simulink library "dhp"  (R2021b)
settings: Solver=VariableStepAuto  StartTime=0.0  StopTime=10.0  RelTol=1e-3
undefined symbols (not defined in the file): ADHP_HysOffset_X_pct, ENUM_POWERSTA_OFF, ENUM_POWERSTA_STANDBY, ENUM_RANGESTA_12IN, ENUM_RANGESTA_12OUT, ENUM_RANGESTA_1OUT, ENUM_RANGESTA_2OUT, ENUM_RESETPEDALZEROPOSREQ_START, FALSE, HUNDRED, KDHP_AcceleratorLoadScalr_gain, KDHP_AccPedalDepressed_pct, KDHP_AccPedalReleased_pct, KDHP_ActAPSPosn_pct_ovrdflg, KDHP_ActAPSPosn_pct_ovrdval, KDHP_DeadBand_pct, KDHP_EAPS11OutWT_gain, KDHP_EAPS12Disagree_pct, KDHP_EAPS12DisagreeTime_s, KDHP_EAPS12OutWT_gain, KDHP_EAPS1AOutWT_gain, KDHP_EAPS1BADHigh_pct, KDHP_EAPS1BADLow_pct, KDHP_EAPS1BADTime_s, KDHP_EAPS1Min_pct_ovrdflg, KDHP_EAPS1Min_pct_ovrdval, KDHP_EAPS1MINInitLowLim_pct, KDHP_EAPS1MINInitUpLim_pct, KDHP_EAPS1WT_gain, KDHP_EAPS21OutWT_gain, KDHP_EAPS22OutWT_gain, KDHP_EAPS2AOutWT_gain, KDHP_EAPS2BADHigh_pct, KDHP_EAPS2BADLow_pct, KDHP_EAPS2BADTime_s, KDHP_EAPS2Min_pct_ovrdflg, KDHP_EAPS2Min_pct_ovrdval, KDHP_EAPS2MINInitLowLim_pct, KDHP_EAPS2MINInitUpLim_pct, KDHP_EAPS2Offset_pct, KDHP_EAPS2Scaler_gain, KDHP_EAPS2WT_gain, KDHP_EAPSCRBadWDSP_pct, KDHP_EAPSLearnDwHigh_pct, KDHP_EAPSLearnDwLow_pct, KDHP_EAPSLearnDwMAX_pct, KDHP_EAPSLearnUpHigh_pct, KDHP_EAPSLearnUpLow_pct, KDHP_EAPSLearnUpOffset_pct, KDHP_EAPSMINLowerLimit_pct, KDHP_EAPSStableThrsh_pct, KDHP_EAPSStableTime_s, KDHP_EPEDPOSNUpLimit_pct, KDHP_GetNRMBaseTime_s, KDHP_LVBattHigh_V, KDHP_LVBattHighLimit_V, KDHP_LVBattLow_V, MDHP_HysOffset_Y_pct, TRUE, ZERO_FLOAT
libraries: hcu_lib x6, simulink x4
(part 1 of 2)
settings Model: Creator=Shawn  LastModifiedBy=FVT23033
settings SolverCC: AlgebraicLoopSolver=TrustRegion

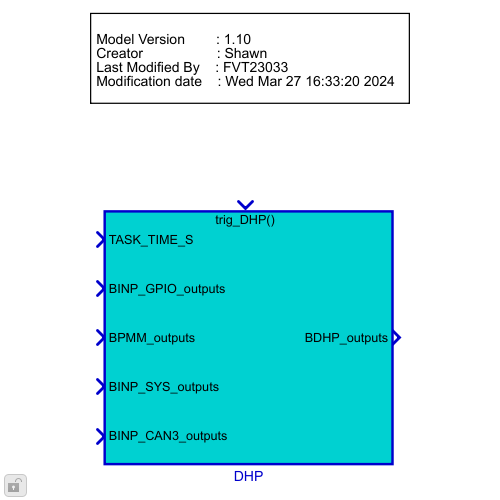
[thumbnail: Simulink's stored preview of the top-level diagram]
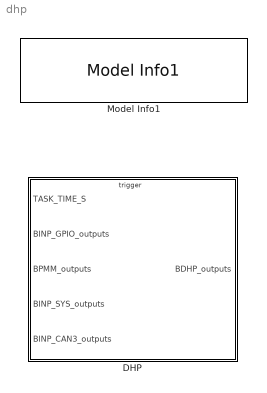
== system dhp ==
  DHP : Subsystem  TreatAsAtomicUnit=on
      settings: RTWSystemCode=Nonreusable function  RTWFcnNameOpts=Use subsystem name  RTWFileNameOpts=Use subsystem name
  Model Info1 : hcu_lib/Model Info1  BlockCM=None  Frame=on  DisplayStringWithTags=|  HorizontalTextAlignment=Left  LeftAlignmentValue=0.02  SourceBlockDiagram=hcu_lib  TagMaxNumber=20
      | Model Version        : %<ModelVersion>
      | Creator                   : %<Creator>
      | Last Modified By    : %<LastModifiedBy>
      | Modification date    : %<LastModificationDate>

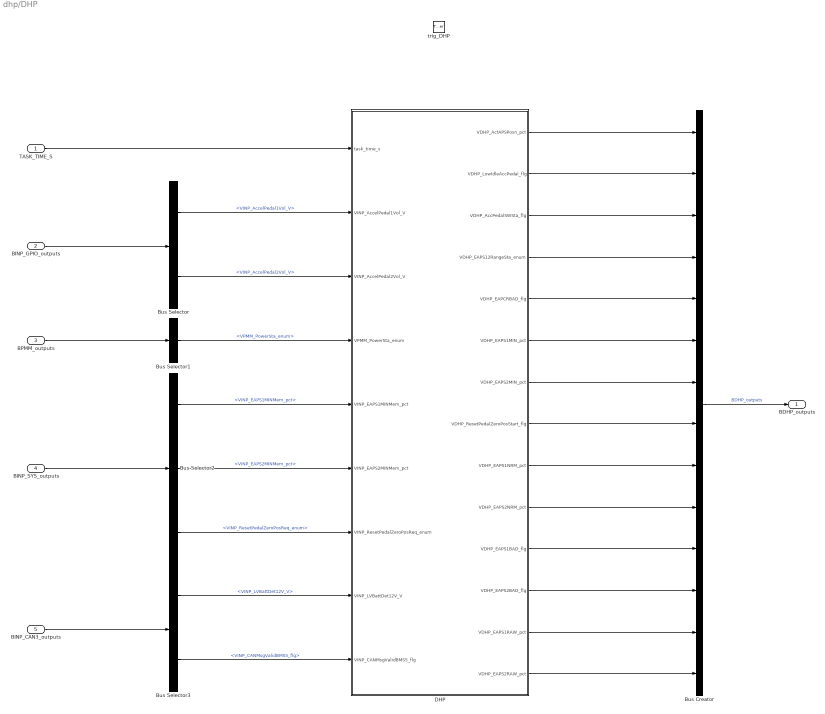
== system dhp/DHP ==
  TASK_TIME_S : Inport
  BINP_GPIO_outputs : Inport  Port=2  OutDataTypeStr=Bus: BINP_GPIO_outputs
  BPMM_outputs : Inport  Port=3  OutDataTypeStr=Bus: BPMM_outputs
  BINP_SYS_outputs : Inport  Port=4  OutDataTypeStr=Bus: BINP_SYS_outputs
  BINP_CAN3_outputs : Inport  Port=5  OutDataTypeStr=Bus: BINP_CAN3_outputs
  trig_DHP : TriggerPort  TriggerType=function-call  VariantControl=(inherit)
  Bus Creator : BusCreator  Inputs=14  OutDataTypeStr=Bus: BDHP_outputs  NonVirtualBus=on
  Bus Selector : BusSelector  OutputSignals=VINP_AccelPedal1Vol_V,VINP_AccelPedal2Vol_V
  Bus Selector1 : BusSelector  OutputSignals=VPMM_PowerSta_enum
  Bus Selector2 : BusSelector  OutputSignals=VINP_EAPS1MINMem_pct,VINP_EAPS2MINMem_pct,VINP_ResetPedalZeroPosReq_enum
  Bus Selector3 : BusSelector  OutputSignals=VINP_LVBattDet12V_V,VINP_CANMsgValidBMS5_flg
  DHP : Subsystem
  BDHP_outputs : Outport  OutDataTypeStr=Bus: BDHP_outputs  VectorParamsAs1DForOutWhenUnconnected=off
  wires:
  Bus Selector/1 -> DHP/2(VINP_AccelPedal1Vol_V)  "<VINP_AccelPedal1Vol_V>"
  BINP_GPIO_outputs/1 -> Bus Selector/1
  TASK_TIME_S/1 -> DHP/1(task_time_s)
  Bus Selector/2 -> DHP/3(VINP_AccelPedal2Vol_V)  "<VINP_AccelPedal2Vol_V>"
  Bus Creator/1 -> BDHP_outputs/1  "BDHP_outputs"
  DHP/1(VDHP_ActAPSPosn_pct) -> Bus Creator/1
  DHP/2(VDHP_LowIdleAccPedal_flg) -> Bus Creator/2
  BPMM_outputs/1 -> Bus Selector1/1
  Bus Selector1/1 -> DHP/4(VPMM_PowerSta_enum)  "<VPMM_PowerSta_enum>"
  DHP/3(VDHP_AccPedalSWSta_flg) -> Bus Creator/3
  DHP/4(VDHP_EAPS12RangeSta_enum) -> Bus Creator/4
  DHP/5(VDHP_EAPCRBAD_flg) -> Bus Creator/5
  DHP/6(VDHP_EAPS1MIN_pct) -> Bus Creator/6
  DHP/7(VDHP_EAPS2MIN_pct) -> Bus Creator/7
  BINP_SYS_outputs/1 -> Bus Selector2/1
  Bus Selector2/1 -> DHP/5(VINP_EAPS1MINMem_pct)  "<VINP_EAPS1MINMem_pct>"
  Bus Selector2/2 -> DHP/6(VINP_EAPS2MINMem_pct)  "<VINP_EAPS2MINMem_pct>"
  BINP_CAN3_outputs/1 -> Bus Selector3/1
  Bus Selector3/1 -> DHP/8(VINP_LVBattDet12V_V)  "<VINP_LVBattDet12V_V>"
  Bus Selector3/2 -> DHP/9(VINP_CANMsgValidBMS5_flg)  "<VINP_CANMsgValidBMS5_flg>"
  Bus Selector2/3 -> DHP/7(VINP_ResetPedalZeroPosReq_enum)  "<VINP_ResetPedalZeroPosReq_enum>"
  DHP/8(VDHP_ResetPedalZeroPosStart_flg) -> Bus Creator/8
  DHP/9(VDHP_EAPS1NRM_pct) -> Bus Creator/9
  DHP/10(VDHP_EAPS2NRM_pct) -> Bus Creator/10
  DHP/11(VDHP_EAPS1BAD_flg) -> Bus Creator/11
  DHP/12(VDHP_EAPS2BAD_flg) -> Bus Creator/12
  DHP/13(VDHP_EAPS1RAW_pct) -> Bus Creator/13
  DHP/14(VDHP_EAPS2RAW_pct) -> Bus Creator/14

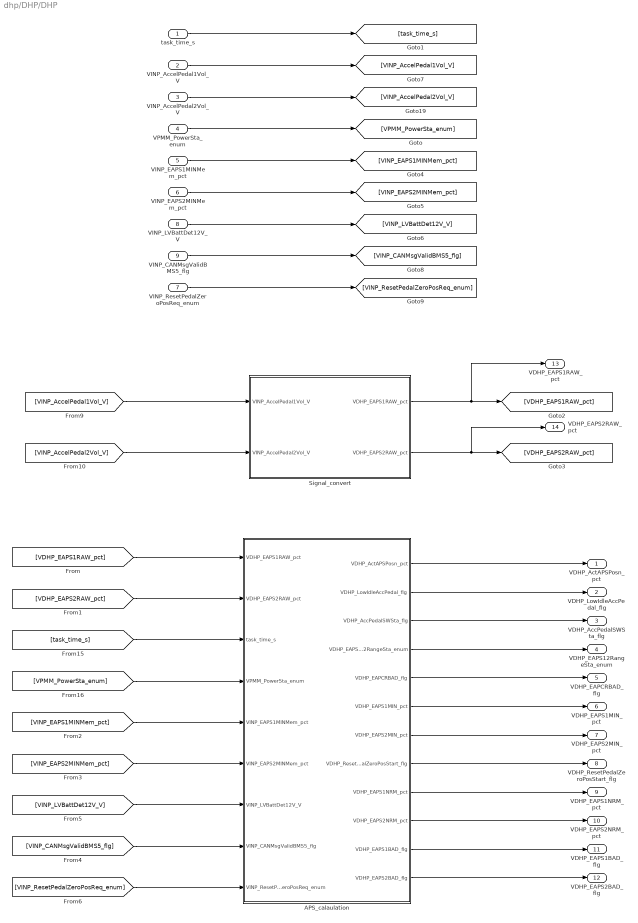
== system dhp/DHP/DHP ==
  task_time_s : Inport
  VINP_AccelPedal1Vol_V : Inport  Port=2
  VINP_AccelPedal2Vol_V : Inport  Port=3
  VPMM_PowerSta_enum : Inport  Port=4
  VINP_EAPS1MINMem_pct : Inport  Port=5
  VINP_EAPS2MINMem_pct : Inport  Port=6
  VINP_ResetPedalZeroPosReq_enum : Inport  Port=7
  VINP_LVBattDet12V_V : Inport  Port=8
  VINP_CANMsgValidBMS5_flg : Inport  Port=9
  APS_calaulation : Subsystem
  Signal_convert : Subsystem
  VDHP_ActAPSPosn_pct : Outport  VectorParamsAs1DForOutWhenUnconnected=off
  VDHP_LowIdleAccPedal_flg : Outport  Port=2  VectorParamsAs1DForOutWhenUnconnected=off
  VDHP_AccPedalSWSta_flg : Outport  Port=3  VectorParamsAs1DForOutWhenUnconnected=off
  VDHP_EAPS12RangeSta_enum : Outport  Port=4  VectorParamsAs1DForOutWhenUnconnected=off
  VDHP_EAPCRBAD_flg : Outport  Port=5  VectorParamsAs1DForOutWhenUnconnected=off
  VDHP_EAPS1MIN_pct : Outport  Port=6  VectorParamsAs1DForOutWhenUnconnected=off
  VDHP_EAPS2MIN_pct : Outport  Port=7  VectorParamsAs1DForOutWhenUnconnected=off
  VDHP_ResetPedalZeroPosStart_flg : Outport  Port=8  VectorParamsAs1DForOutWhenUnconnected=off
  VDHP_EAPS1NRM_pct : Outport  Port=9  VectorParamsAs1DForOutWhenUnconnected=off
  VDHP_EAPS2NRM_pct : Outport  Port=10  VectorParamsAs1DForOutWhenUnconnected=off
  VDHP_EAPS1BAD_flg : Outport  Port=11
  VDHP_EAPS2BAD_flg : Outport  Port=12
  VDHP_EAPS1RAW_pct : Outport  Port=13
  VDHP_EAPS2RAW_pct : Outport  Port=14
  wires:
  VPMM_PowerSta_enum/1 -> [VPMM_PowerSta_enum]
  task_time_s/1 -> [task_time_s]
  VINP_AccelPedal1Vol_V/1 -> [VINP_AccelPedal1Vol_V]
  VINP_AccelPedal2Vol_V/1 -> [VINP_AccelPedal2Vol_V]
  APS_calaulation/1(VDHP_ActAPSPosn_pct) -> VDHP_ActAPSPosn_pct/1
  APS_calaulation/2(VDHP_LowIdleAccPedal_flg) -> VDHP_LowIdleAccPedal_flg/1
  [VPMM_PowerSta_enum] -> APS_calaulation/4(VPMM_PowerSta_enum)
  [VINP_AccelPedal1Vol_V] -> Signal_convert/1(VINP_AccelPedal1Vol_V)
  [VINP_AccelPedal2Vol_V] -> Signal_convert/2(VINP_AccelPedal2Vol_V)
  Signal_convert/1(VDHP_EAPS1RAW_pct) -> VDHP_EAPS1RAW_pct/1, [VDHP_EAPS1RAW_pct]
  [VDHP_EAPS1RAW_pct] -> APS_calaulation/1(VDHP_EAPS1RAW_pct)
  Signal_convert/2(VDHP_EAPS2RAW_pct) -> VDHP_EAPS2RAW_pct/1, [VDHP_EAPS2RAW_pct]
  [VDHP_EAPS2RAW_pct] -> APS_calaulation/2(VDHP_EAPS2RAW_pct)
  APS_calaulation/3(VDHP_AccPedalSWSta_flg) -> VDHP_AccPedalSWSta_flg/1
  APS_calaulation/5(VDHP_EAPCRBAD_flg) -> VDHP_EAPCRBAD_flg/1
  APS_calaulation/4(VDHP_EAPS12RangeSta_enum) -> VDHP_EAPS12RangeSta_enum/1
  [task_time_s] -> APS_calaulation/3(task_time_s)
  APS_calaulation/6(VDHP_EAPS1MIN_pct) -> VDHP_EAPS1MIN_pct/1
  APS_calaulation/7(VDHP_EAPS2MIN_pct) -> VDHP_EAPS2MIN_pct/1
  VINP_EAPS1MINMem_pct/1 -> [VINP_EAPS1MINMem_pct]
  VINP_EAPS2MINMem_pct/1 -> [VINP_EAPS2MINMem_pct]
  [VINP_EAPS1MINMem_pct] -> APS_calaulation/5(VINP_EAPS1MINMem_pct)
  [VINP_EAPS2MINMem_pct] -> APS_calaulation/6(VINP_EAPS2MINMem_pct)
  VINP_CANMsgValidBMS5_flg/1 -> [VINP_CANMsgValidBMS5_flg]
  VINP_LVBattDet12V_V/1 -> [VINP_LVBattDet12V_V]
  [VINP_LVBattDet12V_V] -> APS_calaulation/7(VINP_LVBattDet12V_V)
  [VINP_CANMsgValidBMS5_flg] -> APS_calaulation/8(VINP_CANMsgValidBMS5_flg)
  VINP_ResetPedalZeroPosReq_enum/1 -> [VINP_ResetPedalZeroPosReq_enum]
  [VINP_ResetPedalZeroPosReq_enum] -> APS_calaulation/9(VINP_ResetPedalZeroPosReq_enum)
  APS_calaulation/8(VDHP_ResetPedalZeroPosStart_flg) -> VDHP_ResetPedalZeroPosStart_flg/1
  APS_calaulation/9(VDHP_EAPS1NRM_pct) -> VDHP_EAPS1NRM_pct/1
  APS_calaulation/10(VDHP_EAPS2NRM_pct) -> VDHP_EAPS2NRM_pct/1
  APS_calaulation/12(VDHP_EAPS2BAD_flg) -> VDHP_EAPS2BAD_flg/1
  APS_calaulation/11(VDHP_EAPS1BAD_flg) -> VDHP_EAPS1BAD_flg/1

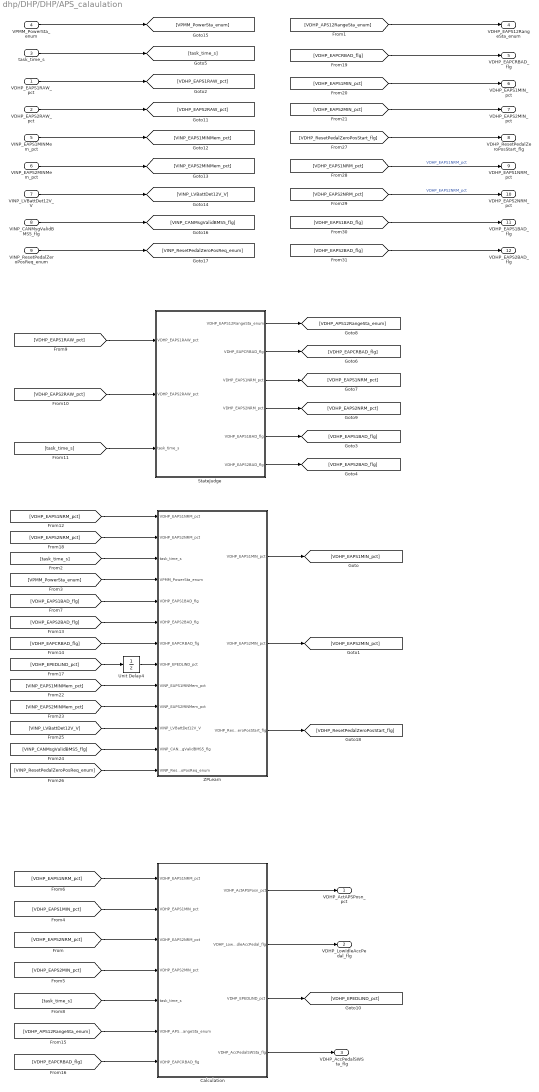
== system dhp/DHP/DHP/APS_calaulation ==
  VDHP_EAPS1RAW_pct : Inport
  VDHP_EAPS2RAW_pct : Inport  Port=2
  task_time_s : Inport  Port=3
  VPMM_PowerSta_enum : Inport  Port=4
  VINP_EAPS1MINMem_pct : Inport  Port=5
  VINP_EAPS2MINMem_pct : Inport  Port=6
  VINP_LVBattDet12V_V : Inport  Port=7
  VINP_CANMsgValidBMS5_flg : Inport  Port=8
  VINP_ResetPedalZeroPosReq_enum : Inport  Port=9
  Calculation : Subsystem
  StateJudge : Subsystem
  Unit Delay4 : UnitDelay  SampleTime=-1  HasFrameUpgradeWarning=on
  ZPLearn : Subsystem
  VDHP_ActAPSPosn_pct : Outport
  VDHP_LowIdleAccPedal_flg : Outport  Port=2
  VDHP_AccPedalSWSta_flg : Outport  Port=3
  VDHP_EAPS12RangeSta_enum : Outport  Port=4
  VDHP_EAPCRBAD_flg : Outport  Port=5
  VDHP_EAPS1MIN_pct : Outport  Port=6
  VDHP_EAPS2MIN_pct : Outport  Port=7
  VDHP_ResetPedalZeroPosStart_flg : Outport  Port=8
  VDHP_EAPS1NRM_pct : Outport  Port=9
  VDHP_EAPS2NRM_pct : Outport  Port=10
  VDHP_EAPS1BAD_flg : Outport  Port=11
  VDHP_EAPS2BAD_flg : Outport  Port=12
  wires:
  [VDHP_EAPS1MIN_pct] -> Calculation/2(VDHP_EAPS1MIN_pct)
  StateJudge/4(VDHP_EAPS2NRM_pct) -> [VDHP_EAPS2NRM_pct]
  [VDHP_EAPS1BAD_flg] -> ZPLearn/5(VDHP_EAPS1BAD_flg)
  [VDHP_EAPS2NRM_pct] -> Calculation/3(VDHP_EAPS2NRM_pct)
  [VDHP_EAPS1RAW_pct] -> StateJudge/1(VDHP_EAPS1RAW_pct)
  VDHP_EAPS2RAW_pct/1 -> [VDHP_EAPS2RAW_pct]
  [VPMM_PowerSta_enum] -> ZPLearn/4(VPMM_PowerSta_enum)
  [task_time_s] -> ZPLearn/3(task_time_s)
  [VDHP_EAPS2MIN_pct] -> Calculation/4(VDHP_EAPS2MIN_pct)
  [task_time_s] -> Calculation/5(task_time_s)
  StateJudge/1(VDHP_EAPS12RangeSta_enum) -> [VDHP_APS12RangeSta_enum]
  [VDHP_EAPS2NRM_pct] -> ZPLearn/2(VDHP_EAPS2NRM_pct)
  VPMM_PowerSta_enum/1 -> [VPMM_PowerSta_enum]
  VDHP_EAPS1RAW_pct/1 -> [VDHP_EAPS1RAW_pct]
  [VDHP_EAPS1NRM_pct] -> ZPLearn/1(VDHP_EAPS1NRM_pct)
  StateJudge/5(VDHP_EAPS1BAD_flg) -> [VDHP_EAPS1BAD_flg]
  [VDHP_EAPS1NRM_pct] -> Calculation/1(VDHP_EAPS1NRM_pct)
  task_time_s/1 -> [task_time_s]
  ZPLearn/2(VDHP_EAPS2MIN_pct) -> [VDHP_EAPS2MIN_pct]
  ZPLearn/1(VDHP_EAPS1MIN_pct) -> [VDHP_EAPS1MIN_pct]
  [VDHP_APS12RangeSta_enum] -> Calculation/6(VDHP_APS12RangeSta_enum)
  [VDHP_EAPCRBAD_flg] -> ZPLearn/7(VDHP_EAPCRBAD_flg)
  [VDHP_EAPS2RAW_pct] -> StateJudge/2(VDHP_EAPS2RAW_pct)
  Calculation/1(VDHP_ActAPSPosn_pct) -> VDHP_ActAPSPosn_pct/1
  [VDHP_EAPCRBAD_flg] -> Calculation/7(VDHP_EAPCRBAD_flg)
  StateJudge/3(VDHP_EAPS1NRM_pct) -> [VDHP_EAPS1NRM_pct]
  StateJudge/2(VDHP_EAPCRBAD_flg) -> [VDHP_EAPCRBAD_flg]
  [VDHP_EAPS2BAD_flg] -> ZPLearn/6(VDHP_EAPS2BAD_flg)
  StateJudge/6(VDHP_EAPS2BAD_flg) -> [VDHP_EAPS2BAD_flg]
  [task_time_s] -> StateJudge/3(task_time_s)
  Calculation/2(VDHP_LowIdleAccPedal_flg) -> VDHP_LowIdleAccPedal_flg/1
  Calculation/3(VDHP_EPEDLIND_pct) -> [VDHP_EPEDLIND_pct]
  [VDHP_EPEDLIND_pct] -> Unit Delay4/1
  Unit Delay4/1 -> ZPLearn/8(VDHP_EPEDLIND_pct)
  Calculation/4(VDHP_AccPedalSWSta_flg) -> VDHP_AccPedalSWSta_flg/1
  [VDHP_EAPCRBAD_flg] -> VDHP_EAPCRBAD_flg/1
  [VDHP_APS12RangeSta_enum] -> VDHP_EAPS12RangeSta_enum/1
  [VDHP_EAPS1MIN_pct] -> VDHP_EAPS1MIN_pct/1
  [VDHP_EAPS2MIN_pct] -> VDHP_EAPS2MIN_pct/1
  VINP_EAPS1MINMem_pct/1 -> [VINP_EAPS1MINMem_pct]
  VINP_EAPS2MINMem_pct/1 -> [VINP_EAPS2MINMem_pct]
  [VINP_EAPS1MINMem_pct] -> ZPLearn/9(VINP_EAPS1MINMem_pct)
  [VINP_EAPS2MINMem_pct] -> ZPLearn/10(VINP_EAPS2MINMem_pct)
  VINP_CANMsgValidBMS5_flg/1 -> [VINP_CANMsgValidBMS5_flg]
  VINP_LVBattDet12V_V/1 -> [VINP_LVBattDet12V_V]
  [VINP_LVBattDet12V_V] -> ZPLearn/11(VINP_LVBattDet12V_V)
  [VINP_CANMsgValidBMS5_flg] -> ZPLearn/12(VINP_CANMsgValidBMS5_flg)
  VINP_ResetPedalZeroPosReq_enum/1 -> [VINP_ResetPedalZeroPosReq_enum]
  [VINP_ResetPedalZeroPosReq_enum] -> ZPLearn/13(VINP_ResetPedalZeroPosReq_enum)
  ZPLearn/3(VDHP_ResetPedalZeroPosStart_flg) -> [VDHP_ResetPedalZeroPosStart_flg]
  [VDHP_ResetPedalZeroPosStart_flg] -> VDHP_ResetPedalZeroPosStart_flg/1
  [VDHP_EAPS1NRM_pct] -> VDHP_EAPS1NRM_pct/1  "VDHP_EAPS1NRM_pct"
  [VDHP_EAPS2NRM_pct] -> VDHP_EAPS2NRM_pct/1  "VDHP_EAPS2NRM_pct"
  [VDHP_EAPS1BAD_flg] -> VDHP_EAPS1BAD_flg/1
  [VDHP_EAPS2BAD_flg] -> VDHP_EAPS2BAD_flg/1

== system dhp/DHP/DHP/Signal_convert ==
  VINP_AccelPedal1Vol_V : Inport
  VINP_AccelPedal2Vol_V : Inport  Port=2
  1-D Lookup Table1 : Lookup_n-D  NumberOfTableDimensions=1  BreakpointsForDimension1=[0 5]  Table=[0 1]  ExtrapMethod=Clip  InternalRulePriority=Speed  RndMeth=Simplest  InputSameDT=on
  1-D Lookup Table4 : Lookup_n-D  NumberOfTableDimensions=1  BreakpointsForDimension1=[0 5]  Table=[0 1]  ExtrapMethod=Clip  InternalRulePriority=Speed  RndMeth=Simplest  InputSameDT=on
  Data Type Conversion : DataTypeConversion  OutDataTypeStr=single
  Data Type Conversion1 : DataTypeConversion  OutDataTypeStr=single
  Gain : Gain  Gain=HUNDRED
  Gain1 : Gain  Gain=HUNDRED
  VDHP_EAPS1RAW_pct : Outport
  VDHP_EAPS2RAW_pct : Outport  Port=2
  wires:
  VINP_AccelPedal1Vol_V/1 -> 1-D Lookup Table4/1
  VINP_AccelPedal2Vol_V/1 -> 1-D Lookup Table1/1
  Gain1/1 -> Data Type Conversion/1
  Data Type Conversion/1 -> VDHP_EAPS1RAW_pct/1  "VDHP_EAPS1RAW_pct"
  1-D Lookup Table4/1 -> Gain1/1
  Data Type Conversion1/1 -> VDHP_EAPS2RAW_pct/1  "VDHP_EAPS2RAW_pct"
  Gain/1 -> Data Type Conversion1/1
  1-D Lookup Table1/1 -> Gain/1

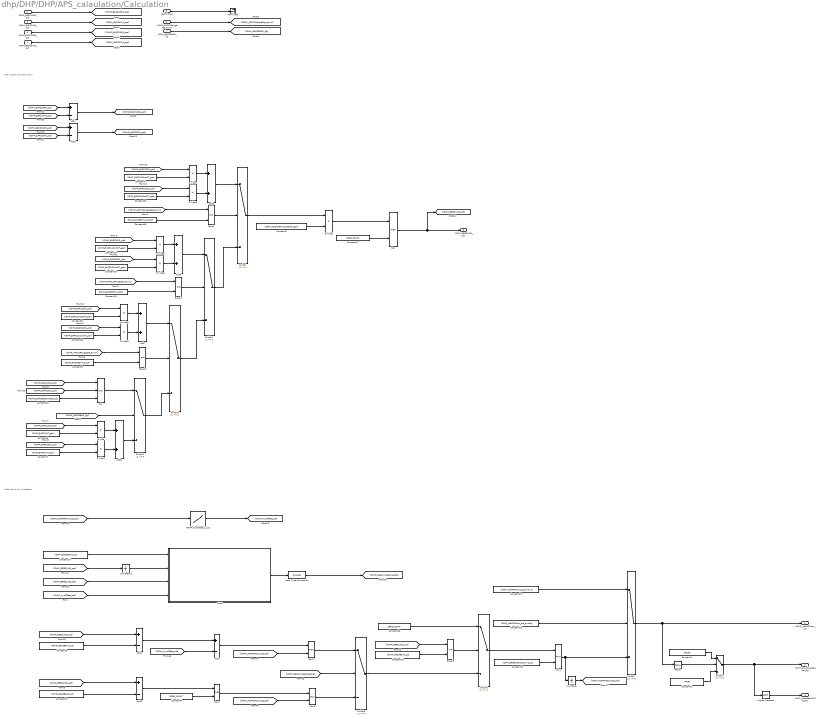
== system dhp/DHP/DHP/APS_calaulation/Calculation ==
  note: Dead band ans Hysteresis
  note: APS weight and calaulation
  VDHP_EAPS1NRM_pct : Inport
  VDHP_EAPS1MIN_pct : Inport  Port=2
  VDHP_EAPS2NRM_pct : Inport  Port=3
  VDHP_EAPS2MIN_pct : Inport  Port=4
  task_time_s : Inport  Port=5
  VDHP_APS12RangeSta_enum : Inport  Port=6
  VDHP_EAPCRBAD_flg : Inport  Port=7
  Add{1..4,6} (5 alike) : Sum  Inputs=+-
  Add{5,7..9} (4 alike) : Sum
  Chart : Stateflow chart  TreatAsAtomicUnit=on
  Constant1 : Constant  Value=FALSE
  Constant{9..10,13..14} (4 alike) : Constant  Value=KDHP_DeadBand_pct
  Constant11 : Constant  Value=ENUM_RANGESTA_1OUT
  Constant12 : Constant  Value=KDHP_EPEDPOSNUpLimit_pct
  Constant15 : Constant  Value=ZERO_FLOAT
  Constant16 : Constant  Value=KDHP_ActAPSPosn_pct_ovrdflg
  Constant17 : Constant  Value=ZERO_FLOAT
  Constant18 : Constant  Value=ENUM_RANGESTA_12OUT
  Constant19 : Constant  Value=KDHP_ActAPSPosn_pct_ovrdval
  Constant2 : Constant  Value=TRUE
  Constant20 : Constant  Value=KDHP_EAPSCRBadWDSP_pct
  Constant21 : Constant  Value=KDHP_EAPS12OutWT_gain
  Constant22 : Constant  Value=KDHP_EAPS22OutWT_gain
  Constant23 : Constant  Value=KDHP_EAPS11OutWT_gain
  Constant24 : Constant  Value=KDHP_EAPS21OutWT_gain
  Constant25 : Constant  Value=KDHP_EAPS2AOutWT_gain
  Constant3 : Constant  Value=KDHP_AcceleratorLoadScalr_gain
  Constant4 : Constant  Value=KDHP_EAPS1AOutWT_gain
  Constant5 : Constant  Value=ENUM_RANGESTA_2OUT
  Constant6 : Constant  Value=KDHP_EAPS1WT_gain
  Constant7 : Constant  Value=KDHP_EAPS2WT_gain
  Constant8 : Constant  Value=ZERO_FLOAT
  Data Type Conversion : DataTypeConversion  OutDataTypeStr=boolean
  Divide{,1..8} (9 alike) : Product  Inputs=**
  Equal : RelationalOperator  Operator===  OutDataTypeStr=boolean  RndMeth=Simplest
  Equal1 : RelationalOperator  Operator===  OutDataTypeStr=boolean  RndMeth=Simplest
  Equal2 : RelationalOperator  Operator===  OutDataTypeStr=boolean  RndMeth=Simplest
  Equal3 : RelationalOperator  Operator=<=  OutDataTypeStr=boolean  RndMeth=Simplest
  Logical Operator : Logic  Operator=NOT  AllPortsSameDT=off  OutDataTypeStr=boolean
  MDHP_HysOffset_Y_pct : Lookup_n-D  NumberOfTableDimensions=1  BreakpointsForDimension1=ADHP_HysOffset_X_pct  Table=MDHP_HysOffset_Y_pct  ExtrapMethod=Clip  InternalRulePriority=Speed  RndMeth=Simplest  InputSameDT=on
  Max : MinMax  Function=max  Inputs=2
  Max2 : MinMax  Function=max  Inputs=2
  Max3 : MinMax  Inputs=2
  Max4 : MinMax  Function=max  Inputs=2
  Min : MinMax  Inputs=3
  Min1 : MinMax  Inputs=2
  Relay : Relay  OnSwitchValue=KDHP_AccPedalDepressed_pct  OffSwitchValue=KDHP_AccPedalReleased_pct
      settings: AttributesFormatString=<ON = %<OnSwitchValue>>\n<OFF = %<OffSwitchValue>>
  Switch{,1..7} (8 alike) : Switch  Criteria=u2 ~= 0
      Switch1 settings: AttributesFormatString=<%<Criteria>>
  Terminator : Terminator
  Unit Delay : UnitDelay  SampleTime=-1  HasFrameUpgradeWarning=on
  Unit Delay1 : UnitDelay  SampleTime=-1  HasFrameUpgradeWarning=on
  VDHP_ActAPSPosn_pct : Outport
  VDHP_LowIdleAccPedal_flg : Outport  Port=2
  VDHP_EPEDLIND_pct : Outport  Port=3
  VDHP_AccPedalSWSta_flg : Outport  Port=4
  wires:
  Max/1 -> VDHP_EPEDLIND_pct/1, [VDHP_EPEDLIND_pct]  "VDHP_EPEDLIND_pct"
  VDHP_EAPS1NRM_pct/1 -> [VDHP_EAPS1NRM_pct]  "VDHP_EAPS1NRM_pct"
  VDHP_EAPS2NRM_pct/1 -> [VDHP_EAPS2NRM_pct]  "VDHP_EAPS2NRM_pct"
  VDHP_EAPS1MIN_pct/1 -> [VDHP_EAPS1MIN_pct]  "VDHP_EAPS1MIN_pct"
  VDHP_EAPS2MIN_pct/1 -> [VDHP_EAPS2MIN_pct]  "VDHP_EAPS2MIN_pct"
  task_time_s/1 -> Terminator/1  "task_time_s"
  VDHP_APS12RangeSta_enum/1 -> [VDHP_APS12RangeSta_enum]  "VDHP_APS12RangeSta_enum"
  VDHP_EAPCRBAD_flg/1 -> [VDHP_EAPCRBAD_flg]  "VDHP_EAPCRBAD_flg"
  Constant2/1 -> Switch1/3
  Switch1/1 -> Logical Operator/1, VDHP_LowIdleAccPedal_flg/1  "VDHP_LowIdleAccPedal_flg"
  Constant1/1 -> Switch1/1
  Relay/1 -> Switch1/2
  Constant3/1 -> Divide2/2
  Equal/1 -> Switch/2
  [VDHP_APS12RangeSta_enum] -> Equal/1
  Constant18/1 -> Equal/2
  Constant11/1 -> Equal1/2
  [VDHP_APS12RangeSta_enum] -> Equal1/1
  Equal1/1 -> Switch2/2
  Switch2/1 -> Switch/3
  [VDHP_EAPS2NRM_pct] -> Add3/1
  [VDHP_EAPS2MIN_pct] -> Add3/2
  Add3/1 -> [VDHP_EAPS2DIS_pct]  "VDHP_EAPS2DIS_pct"
  [VDHP_EAPS1NRM_pct] -> Add4/1
  Add4/1 -> [VDHP_EAPS1DIS_pct]  "VDHP_EAPS1DIS_pct"
  [VDHP_EAPS1MIN_pct] -> Add4/2
  Switch3/1 -> Switch2/3
  [VDHP_APS12RangeSta_enum] -> Equal2/1
  Constant5/1 -> Equal2/2
  Equal2/1 -> Switch3/2
  Switch4/1 -> Switch3/3
  [VDHP_EAPCRBAD_flg] -> Switch4/2
  Min/1 -> Switch4/1
  [VDHP_EAPS2DIS_pct] -> Min/2
  [VDHP_EAPS1DIS_pct] -> Min/1
  [VDHP_EAPS2DIS_pct] -> Divide1/1
  Divide1/1 -> Add5/2
  Divide/1 -> Add5/1
  Add5/1 -> Switch4/3
  [VDHP_EAPS1DIS_pct] -> Divide/1
  Constant6/1 -> Divide/2
  Constant7/1 -> Divide1/2
  Switch/1 -> Divide2/1  "VDHP_EAPSWDSP_pct"
  Constant12/1 -> Min1/2
  Switch7/1 -> VDHP_ActAPSPosn_pct/1, Relay/1  "VDHP_ActAPSPosn_pct"
  Divide2/1 -> Max/1
  Constant17/1 -> Max/2
  [VDHP_ActAPSPosnLast_pct] -> MDHP_HysOffset_Y_pct/1
  [VDHP_PedalIncreasing_flg] -> Switch5/2
  MDHP_HysOffset_Y_pct/1 -> [VDHP_HysOffset_pct]  "VDHP_HysOffset_pct"
  [VDHP_EPEDLIND_pct] -> Add1/1
  [VDHP_ActAPSPosnLast_pct] -> Max2/2
  Max2/1 -> Switch5/1
  Max4/1 -> Max3/1
  [VDHP_HysOffset_pct] -> Add2/2
  Add2/1 -> Max2/1
  [VDHP_ActAPSPosnLast_pct] -> Max3/2
  Max3/1 -> Switch5/3
  Add1/1 -> Add2/1
  [VDHP_EPEDLIND_pct] -> Add6/1
  Constant13/1 -> Add6/2
  Constant8/1 -> Max4/2
  Constant9/1 -> Add1/2
  Add6/1 -> Max4/1
  Unit Delay1/1 -> Chart/2(VDHP_EPEDLINDLast_pct)
  [VDHP_EPEDLIND_pct] -> Unit Delay1/1
  Chart/1(VDHP_PedalIncreasing_flg) -> Data Type Conversion/1
  Constant14/1 -> Chart/1(KDHP_DeadBand_pct)
  [VDHP_HysOffset_pct] -> Chart/4(VDHP_HysOffset_pct)
  [VDHP_EPEDLIND_pct] -> Chart/3(VDHP_EPEDLIND_pct)
  Data Type Conversion/1 -> [VDHP_PedalIncreasing_flg]  "VDHP_PedalIncreasing_flg"
  Switch5/1 -> Switch6/3
  Constant10/1 -> Equal3/2
  [VDHP_EPEDLIND_pct] -> Equal3/1
  Equal3/1 -> Switch6/2
  Constant15/1 -> Switch6/1
  Switch6/1 -> Min1/1
  Logical Operator/1 -> VDHP_AccPedalSWSta_flg/1  "VDHP_AccPedalSWSta_flg"
  Min1/1 -> Unit Delay/1, Switch7/3
  Constant16/1 -> Switch7/2
  Constant19/1 -> Switch7/1
  Unit Delay/1 -> [VDHP_ActAPSPosnLast_pct]
  Constant20/1 -> Min/3
  [VDHP_EAPS2DIS_pct] -> Divide4/1
  Constant22/1 -> Divide4/2
  Constant21/1 -> Divide3/2
  [VDHP_EAPS1DIS_pct] -> Divide3/1
  Divide4/1 -> Add7/2
  Divide3/1 -> Add7/1
  Add7/1 -> Switch3/1
  Divide5/1 -> Add8/1
  Constant24/1 -> Divide6/2
  Constant23/1 -> Divide5/2
  [VDHP_EAPS2DIS_pct] -> Divide6/1
  Divide6/1 -> Add8/2
  [VDHP_EAPS1DIS_pct] -> Divide5/1
  Add8/1 -> Switch2/1
  Add9/1 -> Switch/1
  [VDHP_EAPS1DIS_pct] -> Divide7/1
  [VDHP_EAPS2DIS_pct] -> Divide8/1
  Constant25/1 -> Divide8/2
  Constant4/1 -> Divide7/2
  Divide8/1 -> Add9/2
  Divide7/1 -> Add9/1

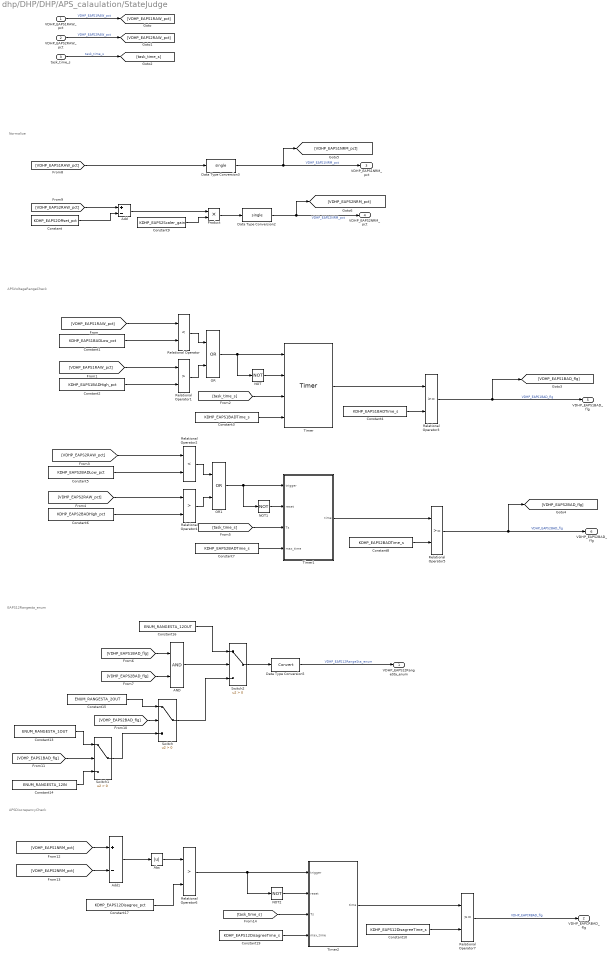
== system dhp/DHP/DHP/APS_calaulation/StateJudge ==
  note: APSDiscrepancyCheck
  note: EAPS12Rangesta_enum
  note: Normalize
  note: APSVoltageRangeCheck
  VDHP_EAPS1RAW_pct : Inport
  VDHP_EAPS2RAW_pct : Inport  Port=2
  task_time_s : Inport  Port=3
  AND : Logic  AllPortsSameDT=off  OutDataTypeStr=boolean
  Abs : Abs
  Add : Sum  Inputs=+-
  Add1 : Sum  Inputs=+-
  Constant : Constant  Value=KDHP_EAPS2Offset_pct
  Constant1 : Constant  Value=KDHP_EAPS1BADLow_pct
  Constant10 : Constant  Value=KDHP_EAPS12DisagreeTime_s
  Constant13 : Constant  Value=ENUM_RANGESTA_1OUT
  Constant14 : Constant  Value=ENUM_RANGESTA_12IN
  Constant15 : Constant  Value=ENUM_RANGESTA_2OUT
  Constant16 : Constant  Value=ENUM_RANGESTA_12OUT
  Constant17 : Constant  Value=KDHP_EAPS12Disagree_pct
  Constant19 : Constant  Value=KDHP_EAPS12DisagreeTime_s
  Constant2 : Constant  Value=KDHP_EAPS1BADHigh_pct
  Constant3 : Constant  Value=KDHP_EAPS1BADTime_s
  Constant4 : Constant  Value=KDHP_EAPS1BADTime_s
  Constant5 : Constant  Value=KDHP_EAPS2BADLow_pct
  Constant6 : Constant  Value=KDHP_EAPS2BADHigh_pct
  Constant7 : Constant  Value=KDHP_EAPS2BADTime_s
  Constant8 : Constant  Value=KDHP_EAPS2BADTime_s
  Constant9 : Constant  Value=KDHP_EAPS2Scaler_gain
  Data Type Conversion2 : DataTypeConversion  OutDataTypeStr=single
  Data Type Conversion3 : DataTypeConversion  OutDataTypeStr=single
  Data Type Conversion5 : DataTypeConversion
  NOT : Logic  Operator=NOT  AllPortsSameDT=off  OutDataTypeStr=boolean
  NOT1 : Logic  Operator=NOT  AllPortsSameDT=off  OutDataTypeStr=boolean
  NOT2 : Logic  Operator=NOT  AllPortsSameDT=off  OutDataTypeStr=boolean
  OR : Logic  Operator=OR  AllPortsSameDT=off  OutDataTypeStr=boolean
  OR1 : Logic  Operator=OR  AllPortsSameDT=off  OutDataTypeStr=boolean
  Product : Product
  Relational Operator : RelationalOperator  Operator=<  OutDataTypeStr=boolean  RndMeth=Simplest
  Relational Operator1 : RelationalOperator  Operator=>  OutDataTypeStr=boolean  RndMeth=Simplest
  Relational Operator2 : RelationalOperator  Operator=<  OutDataTypeStr=boolean  RndMeth=Simplest
  Relational Operator3 : RelationalOperator  OutDataTypeStr=boolean  RndMeth=Simplest
  Relational Operator4 : RelationalOperator  Operator=>  OutDataTypeStr=boolean  RndMeth=Simplest
  Relational Operator5 : RelationalOperator  OutDataTypeStr=boolean  RndMeth=Simplest
  Relational Operator6 : RelationalOperator  Operator=>  OutDataTypeStr=boolean  RndMeth=Simplest
  Relational Operator7 : RelationalOperator  OutDataTypeStr=boolean  RndMeth=Simplest
  Switch : Switch  Criteria=u2 > Threshold
  Switch1 : Switch  Criteria=u2 > Threshold
  Switch2 : Switch  Criteria=u2 > Threshold
  Timer : hcu_lib/Basic_Blocks/Timer
  Timer1 : Subsystem  mask(Timer){}
      mask help: Timer funcion.
  Timer2 : Subsystem  mask(Timer){}
      mask help: Timer funcion.
  VDHP_EAPS12RangeSta_enum : Outport
  VDHP_EAPCRBAD_flg : Outport  Port=2
  VDHP_EAPS1NRM_pct : Outport  Port=3
  VDHP_EAPS2NRM_pct : Outport  Port=4
  VDHP_EAPS1BAD_flg : Outport  Port=5
  VDHP_EAPS2BAD_flg : Outport  Port=6
  wires:
  Relational Operator1/1 -> OR/2
  [VDHP_EAPS1RAW_pct] -> Relational Operator1/1
  Relational Operator/1 -> OR/1
  VDHP_EAPS1RAW_pct/1 -> [VDHP_EAPS1RAW_pct]  "VDHP_EAPS1RAW_pct"
  [VDHP_EAPS1RAW_pct] -> Relational Operator/1
  VDHP_EAPS2RAW_pct/1 -> [VDHP_EAPS2RAW_pct]  "VDHP_EAPS2RAW_pct"
  task_time_s/1 -> [task_time_s]  "task_time_s"
  OR/1 -> NOT/1, Timer/1
  NOT/1 -> Timer/2
  Constant4/1 -> Relational Operator3/2
  Relational Operator3/1 -> VDHP_EAPS1BAD_flg/1, [VDHP_EAPS1BAD_flg]  "VDHP_EAPS1BAD_flg"
  Relational Operator5/1 -> VDHP_EAPS2BAD_flg/1, [VDHP_EAPS2BAD_flg]  "VDHP_EAPS2BAD_flg"
  Constant8/1 -> Relational Operator5/2
  OR1/1 -> Timer1/1(trigger), NOT1/1
  [VDHP_EAPS2RAW_pct] -> Relational Operator2/1
  Relational Operator2/1 -> OR1/1
  Constant5/1 -> Relational Operator2/2
  [VDHP_EAPS2RAW_pct] -> Relational Operator4/1
  Constant6/1 -> Relational Operator4/2
  Relational Operator4/1 -> OR1/2
  Constant1/1 -> Relational Operator/2
  Constant2/1 -> Relational Operator1/2
  [VDHP_EAPS1BAD_flg] -> AND/1
  [VDHP_EAPS2BAD_flg] -> AND/2
  Constant/1 -> Add/2
  Data Type Conversion2/1 -> [VDHP_EAPS2NRM_pct], VDHP_EAPS2NRM_pct/1  "VDHP_EAPS2NRM_pct"
  [VDHP_EAPS2BAD_flg] -> Switch/2
  Switch1/1 -> Switch/3
  [VDHP_EAPS1BAD_flg] -> Switch1/2
  AND/1 -> Switch2/2
  Switch/1 -> Switch2/3
  Constant13/1 -> Switch1/1
  Constant14/1 -> Switch1/3
  Constant15/1 -> Switch/1
  Switch2/1 -> Data Type Conversion5/1
  Constant16/1 -> Switch2/1
  [VDHP_EAPS1RAW_pct] -> Data Type Conversion3/1
  Data Type Conversion3/1 -> [VDHP_EAPS1NRM_pct], VDHP_EAPS1NRM_pct/1  "VDHP_EAPS1NRM_pct"
  [VDHP_EAPS1NRM_pct] -> Add1/1
  [VDHP_EAPS2NRM_pct] -> Add1/2
  Add1/1 -> Abs/1
  Abs/1 -> Relational Operator6/1
  Constant17/1 -> Relational Operator6/2
  Data Type Conversion5/1 -> VDHP_EAPS12RangeSta_enum/1  "VDHP_EAPS12RangeSta_enum"
  [VDHP_EAPS2RAW_pct] -> Add/1
  Add/1 -> Product/1
  Product/1 -> Data Type Conversion2/1
  Constant9/1 -> Product/2
  [task_time_s] -> Timer/3
  Timer/1 -> Relational Operator3/1
  Constant3/1 -> Timer/4
  NOT1/1 -> Timer1/2(reset)
  [task_time_s] -> Timer1/3(Ts)
  Constant7/1 -> Timer1/4(max_time)
  Timer1/1(time) -> Relational Operator5/1
  Relational Operator6/1 -> NOT2/1, Timer2/1(trigger)
  NOT2/1 -> Timer2/2(reset)
  [task_time_s] -> Timer2/3(Ts)
  Constant19/1 -> Timer2/4(max_time)
  Timer2/1(time) -> Relational Operator7/1
  Constant10/1 -> Relational Operator7/2
  Relational Operator7/1 -> VDHP_EAPCRBAD_flg/1  "VDHP_EAPCRBAD_flg"

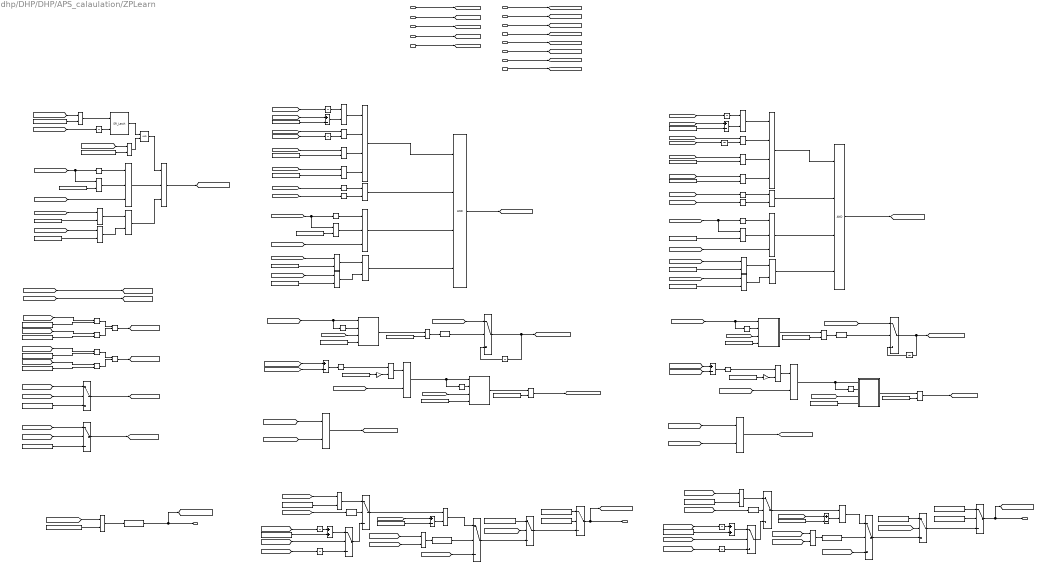
== system dhp/DHP/DHP/APS_calaulation/ZPLearn ==
  note: EAPS1 ZP update
  note: use real pedal position percentage,
      | not NRM percentage
  note: APS learn up judgement
  note: use real pedal position percentage,
      | not NRM percentage
  note: EAPS2 learn down judgement
  note: EAPS1 learn down judgement
  note: APS initial value
  note: EAPS2 ZP update
  note: Reset Pedal Zero Pos Request
  VDHP_EAPS1NRM_pct : Inport
  VDHP_EAPS2NRM_pct : Inport  Port=2
  task_time_s : Inport  Port=3
  VPMM_PowerSta_enum : Inport  Port=4
  VDHP_EAPS1BAD_flg : Inport  Port=5
  VDHP_EAPS2BAD_flg : Inport  Port=6
  VDHP_EAPCRBAD_flg : Inport  Port=7
  VDHP_EPEDLIND_pct : Inport  Port=8
  VINP_EAPS1MINMem_pct : Inport  Port=9
  VINP_EAPS2MINMem_pct : Inport  Port=10
  VINP_LVBattDet12V_V : Inport  Port=11
  VINP_CANMsgValidBMS5_flg : Inport  Port=12
  VINP_ResetPedalZeroPosReq_enum : Inport  Port=13
  AND{,1..4,6..7,10,13..14} (10 alike) : Logic  AllPortsSameDT=off  OutDataTypeStr=boolean
  AND{5,9,11..12} (4 alike) : Logic  Inputs=3  AllPortsSameDT=off  OutDataTypeStr=boolean
  AND15 : Logic  Inputs=4  AllPortsSameDT=off  OutDataTypeStr=boolean
  AND16 : Logic  Operator=OR  AllPortsSameDT=off  OutDataTypeStr=boolean
  AND17 : Logic  Operator=OR  AllPortsSameDT=off  OutDataTypeStr=boolean
  AND8 : Logic  Inputs=4  AllPortsSameDT=off  OutDataTypeStr=boolean
  Abs : Abs
  Abs1 : Abs
  Add{1..4,7..8} (6 alike) : Sum  Inputs=+-
  Add5 : Sum
  Add6 : Sum
  Constant1 : Constant  Value=KDHP_EAPSLearnDwLow_pct
  Constant{9..10,25,33} (4 alike) : Constant  Value=KDHP_EAPSStableTime_s
  Constant11 : Constant  Value=KDHP_EAPSLearnDwLow_pct
  Constant{2,12,17,42..44} (6 alike) : Constant  Value=KDHP_EAPSLearnDwHigh_pct
  Constant{3,13,21..22} (4 alike) : Constant  Value=KDHP_EAPSLearnDwMAX_pct
  Constant14 : Constant  Value=KDHP_EAPS2Min_pct_ovrdflg
  Constant15 : Constant  Value=KDHP_EAPS2Min_pct_ovrdval
  Constant16 : Constant  Value=KDHP_EAPSLearnUpOffset_pct
  Constant18 : Constant  Value=KDHP_EAPSStableThrsh_pct
  Constant{7..8,19..20} (4 alike) : Constant  Value=KDHP_GetNRMBaseTime_s
  Constant23 : Constant  Value=KDHP_LVBattHighLimit_V
  Constant24 : Constant  Value=ENUM_POWERSTA_OFF
  Constant26 : Constant  Value=ENUM_POWERSTA_STANDBY
  Constant27 : Constant  Value=KDHP_LVBattHighLimit_V
  Constant28 : Constant  Value=ENUM_POWERSTA_OFF
  Constant29 : Constant  Value=ENUM_POWERSTA_STANDBY
  Constant30 : Constant  Value=KDHP_LVBattHighLimit_V
  Constant31 : Constant  Value=ENUM_POWERSTA_OFF
  Constant32 : Constant  Value=ENUM_POWERSTA_STANDBY
  Constant34 : Constant  Value=ENUM_RESETPEDALZEROPOSREQ_START
  Constant35 : Constant  Value=KDHP_EAPSLearnUpLow_pct
  Constant36 : Constant  Value=KDHP_EAPS1MINInitUpLim_pct  VectorParams1D=off
  Constant37 : Constant  Value=KDHP_EAPS2MINInitUpLim_pct  VectorParams1D=off
  Constant38 : Constant  Value=KDHP_EAPS2MINInitLowLim_pct  VectorParams1D=off
  Constant39 : Constant  Value=KDHP_EAPS1Min_pct_ovrdflg
  Constant4 : Constant  Value=KDHP_EAPS1MINInitLowLim_pct  VectorParams1D=off
  Constant40 : Constant  Value=KDHP_EAPS1Min_pct_ovrdval
  Constant41 : Constant  Value=KDHP_EAPSLearnUpOffset_pct
  Constant45 : Constant  Value=KDHP_EAPSMINLowerLimit_pct
  Constant46 : Constant  Value=KDHP_EAPSMINLowerLimit_pct
  Constant5 : Constant  Value=KDHP_EAPSLearnUpHigh_pct
  Constant6 : Constant  Value=KDHP_EAPSStableThrsh_pct
  Detect Increase{1..4} (4 alike) : simulink/Logic and Bit Operations/Detect Increase  vinit=0.0  OutDataTypeStr=boolean
  Gain : Gain  Gain=0.5
  Gain1 : Gain  Gain=0.5
  Latch : hcu_lib/Basic_Blocks/Latch
  Latch1 : hcu_lib/Basic_Blocks/Latch
  Latch2 : hcu_lib/Basic_Blocks/Latch
  Logical Operator2 : Logic  AllPortsSameDT=off  OutDataTypeStr=boolean
  Logical Operator3 : Logic  AllPortsSameDT=off  OutDataTypeStr=boolean
  Max{,1..3} (4 alike) : MinMax  Function=max  Inputs=2
  NOT{,1..7} (8 alike) : Logic  Operator=NOT  AllPortsSameDT=off  OutDataTypeStr=boolean
  OR1 : Logic  Inputs=4  AllPortsSameDT=off  OutDataTypeStr=boolean
  OR4 : Logic  Inputs=4  AllPortsSameDT=off  OutDataTypeStr=boolean
  Relational Operator{,3..5,9,20..21,24,26} (9 alike) : RelationalOperator  OutDataTypeStr=boolean  RndMeth=Simplest
  Relational Operator{1..2,6,10,15..16,19,22..23,25} (10 alike) : RelationalOperator  Operator=<=  OutDataTypeStr=boolean  RndMeth=Simplest
  Relational Operator{11,14,17..18,27..28} (6 alike) : RelationalOperator  Operator=~=  OutDataTypeStr=boolean  RndMeth=Simplest
  Relational Operator12 : RelationalOperator  Operator=>  OutDataTypeStr=boolean  RndMeth=Simplest
  Relational Operator13 : RelationalOperator  Operator=<  OutDataTypeStr=boolean  RndMeth=Simplest
  Relational Operator29 : RelationalOperator  Operator===  OutDataTypeStr=boolean  RndMeth=Simplest
  Relational Operator7 : RelationalOperator  Operator=>  OutDataTypeStr=boolean  RndMeth=Simplest
  Relational Operator8 : RelationalOperator  Operator=<  OutDataTypeStr=boolean  RndMeth=Simplest
  Relay : Relay  OnSwitchValue=KDHP_LVBattHigh_V  OffSwitchValue=KDHP_LVBattLow_V  OutDataTypeStr=boolean
      settings: AttributesFormatString=|
      | ON: %<OnSwitchValue>
      | OFF: %<OffSwitchValue>
  Relay1 : Relay  OnSwitchValue=KDHP_LVBattHigh_V  OffSwitchValue=KDHP_LVBattLow_V  OutDataTypeStr=boolean
      settings: AttributesFormatString=|
      | ON: %<OnSwitchValue>
      | OFF: %<OffSwitchValue>
  Relay2 : Relay  OnSwitchValue=KDHP_LVBattHigh_V  OffSwitchValue=KDHP_LVBattLow_V  OutDataTypeStr=boolean
      settings: AttributesFormatString=|
      | ON: %<OnSwitchValue>
      | OFF: %<OffSwitchValue>
  SR_Latch : hcu_lib/Basic_Blocks/SR_Latch
  Switch : Switch  Criteria=u2 > Threshold
  Switch{1..8,17..20,22} (13 alike) : Switch  Criteria=u2 ~= 0
  Timer1 : Subsystem  mask(Timer){}
      mask help: Timer funcion.
  Timer2 : Subsystem  mask(Timer){}
      mask help: Timer funcion.
  Timer3 : Subsystem  mask(Timer){}
      mask help: Timer funcion.
  Timer4 : Subsystem  mask(Timer){}
      mask help: Timer funcion.
  Unit Delay{1..2,4,6,9..14,17} (11 alike) : UnitDelay  SampleTime=-1  HasFrameUpgradeWarning=on
  VDHP_EAPS1MIN_pct : Outport
  VDHP_EAPS2MIN_pct : Outport  Port=2
  VDHP_ResetPedalZeroPosStart_flg : Outport  Port=3
  wires:
  Relational Operator23/1 -> Logical Operator2/1
  [VDHP_EAPS1MINMem_pct] -> Relational Operator23/1
  Constant4/1 -> Relational Operator24/2
  [VDHP_EAPSLearnUpEnable_flg] -> Unit Delay12/1
  [VDHP_EAPS1MINMem_pct] -> Relational Operator24/1
  Constant36/1 -> Relational Operator23/2
  AND4/1 -> [VDHP_EAPS2LearnDwEnable_flg]  "VDHP_EAPS2LearnDwEnable_flg"
  Unit Delay6/1 -> Switch6/3
  Constant14/1 -> Switch2/2
  [VDHP_EAPS1LearnInRange_flg] -> NOT4/1, Timer3/1(trigger)
  [task_time_s] -> Timer1/3(Ts)
  Constant7/1 -> Timer2/4(max_time)
  [task_time_s] -> Timer3/3(Ts)
  Constant12/1 -> Relational Operator6/2
  Unit Delay1/1 -> Switch1/3
  Constant19/1 -> Relational Operator9/2
  Detect Increase4/1 -> Switch6/2
  Gain/1 -> Relational Operator15/2
  Timer2/1(time) -> Relational Operator3/1
  Constant9/1 -> Timer4/4(max_time)
  AND/1 -> AND11/1
  Detect Increase2/1 -> Switch3/2
  NOT4/1 -> Timer3/2(reset)
  Constant20/1 -> Timer3/4(max_time)
  NOT1/1 -> Timer2/2(reset)
  [VDHP_EAPS2NRM_pct] -> Switch1/1
  Constant8/1 -> Relational Operator3/2
  Relational Operator4/1 -> [VDHP_EAPS2NRMStable_flg]  "VDHP_EAPS2NRMStable_flg"
  [VDHP_EAPS2MIN_pct] -> Unit Delay10/1
  [task_time_s] -> Timer2/3(Ts)
  Unit Delay12/1 -> SR_Latch/2
  [VDHP_EAPS2NRMBase_pct] -> Add3/2
  Switch1/1 -> Unit Delay1/1, [VDHP_EAPS2NRMBase_pct]
  Relational Operator3/1 -> Detect Increase3/1
  [VDHP_EAPS2BAD_flg] -> NOT6/1
  Timer3/1(time) -> Relational Operator9/1
  [VDHP_EAPS2NRM_pct] -> Relational Operator8/1
  [VDHP_EAPCRBAD_flg] -> NOT7/1
  VDHP_EAPS1NRM_pct/1 -> [VDHP_EAPS1NRM_pct]
  Add4/1 -> Relational Operator7/2
  Unit Delay9/1 -> Relational Operator7/1
  VDHP_EAPCRBAD_flg/1 -> [VDHP_EAPCRBAD_flg]
  Constant11/1 -> Relational Operator5/2
  OR1/1 -> [VDHP_EAPS2LearnInRange_flg]  "VDHP_EAPS2LearnInRange_flg"
  AND3/1 -> NOT3/1, Timer4/1(trigger)
  [VDHP_EAPS1BAD_flg] -> NOT/1
  Timer4/1(time) -> Relational Operator4/1
  Logical Operator2/1 -> [VDHP_EAPS1MINMemValid_flg]
  [VDHP_EAPS2MIN_pct] -> Unit Delay11/1
  Constant13/1 -> Add4/2
  [VDHP_EAPS2MINInit_pct] -> Add4/1
  Add3/1 -> Abs1/1
  Relational Operator2/1 -> AND3/1
  [VDHP_EAPS1NRM_pct] -> Relational Operator1/1
  Constant1/1 -> Relational Operator/2
  [VDHP_EAPS2NRMStable_flg] -> AND4/2
  Constant6/1 -> Gain1/1
  Constant2/1 -> Relational Operator1/2
  [VDHP_EAPS2LearnDwEnable_flg] -> Detect Increase2/1
  [VDHP_EAPS1NRM_pct] -> Relational Operator13/1
  Gain1/1 -> Relational Operator2/2
  [VDHP_EAPS1NRM_pct] -> Relational Operator/1
  AND2/1 -> [VDHP_EAPS1LearnDwEnable_flg]  "VDHP_EAPS1LearnDwEnable_flg"
  [VDHP_EAPS1MIN_pct] -> Unit Delay17/1
  Unit Delay4/1 -> Relational Operator13/2
  [VDHP_EAPS2MINMem_pct] -> Relational Operator26/1
  Constant5/1 -> Relational Operator21/2
  Constant3/1 -> Add1/2
  Switch2/1 -> VDHP_EAPS2MIN_pct/1, [VDHP_EAPS2MIN_pct]  "VDHP_EAPS2MIN_pct"
  [VDHP_EAPS1MIN_pct] -> Unit Delay4/1
  AND1/1 -> NOT5/1, Timer1/1(trigger)
  [VDHP_EAPS1NRMStable_flg] -> AND2/2
  Add1/1 -> Relational Operator12/2
  Constant18/1 -> Gain/1
  [VDHP_EAPS1NRM_pct] -> Add2/1
  Abs1/1 -> Relational Operator2/1  "VDHP_EAPS2NRMDiff_pct"
  Add6/1 -> Switch4/1
  Abs/1 -> Relational Operator15/1  "VDHP_EAPS1NRMDiff_pct"
  Add2/1 -> Abs/1
  Add5/1 -> Switch19/1
  Relational Operator9/1 -> Detect Increase4/1
  Relational Operator15/1 -> AND1/1
  [VDHP_EAPS1LearnInRange_flg] -> AND1/2
  [VDHP_EAPS2NRM_pct] -> Relational Operator6/1
  Switch20/1 -> Switch17/3
  Latch1/1 -> Switch5/2  "VDHP_EAPS2Learned_flg"
  [VDHP_EAPS1MINInit_pct] -> Add1/1
  NOT3/1 -> Timer4/2(reset)
  [task_time_s] -> Timer4/3(Ts)
  Constant15/1 -> Switch2/1
  Unit Delay17/1 -> Switch19/3
  [VDHP_EAPCRBAD_flg] -> NOT2/1
  [VDHP_EAPS1LearnDwEnable_flg] -> Detect Increase1/1
  Constant35/1 -> Relational Operator22/2
  Detect Increase3/1 -> Switch1/2
  Constant10/1 -> Relational Operator4/2
  Relational Operator24/1 -> Logical Operator2/2
  Logical Operator3/1 -> [VDHP_EAPS2MINMemValid_flg]
  [VDHP_EAPS2MINMem_pct] -> Relational Operator25/1
  [VDHP_EAPS2LearnInRange_flg] -> AND3/2
  Detect Increase1/1 -> Switch18/2
  Switch19/1 -> Switch18/3
  Unit Delay14/1 -> Add5/1
  Constant41/1 -> Add5/2
  [VDHP_EAPS1MIN_pct] -> Unit Delay14/1
  Relational Operator25/1 -> Logical Operator3/1
  Constant38/1 -> Relational Operator26/2
  Relational Operator26/1 -> Logical Operator3/2
  Unit Delay10/1 -> Relational Operator8/2
  VDHP_EAPS1BAD_flg/1 -> [VDHP_EAPS1BAD_flg]
  [VDHP_EAPSLearnUpEnable_flg] -> Switch4/2
  [VDHP_EAPS2NRM_pct] -> Relational Operator5/1
  [VDHP_EAPSLearnUpEnable_flg] -> Switch19/2
  OR4/1 -> [VDHP_EAPS1LearnInRange_flg]  "VDHP_EAPS1LearnInRange_flg"
  Switch4/1 -> Switch3/3
  Constant16/1 -> Add6/2
  [VDHP_EAPS1NRM_pct] -> Switch6/1
  Constant37/1 -> Relational Operator25/2
  Unit Delay11/1 -> Add6/1
  Unit Delay2/1 -> Relational Operator12/1
  task_time_s/1 -> [task_time_s]
  [VDHP_EPEDLIND_pct] -> Relational Operator21/1
  Relational Operator22/1 -> AND/2
  Unit Delay13/1 -> Switch4/3
  [VDHP_EPEDLIND_pct] -> Relational Operator22/1
  Relational Operator21/1 -> SR_Latch/1
  [VDHP_EAPS2LearnInRange_flg] -> NOT1/1, Timer2/1(trigger)
  Constant25/1 -> Timer1/4(max_time)
  [VDHP_EAPS2MIN_pct] -> Unit Delay13/1
  Switch6/1 -> Unit Delay6/1, [VDHP_EAPS1NRMBase_pct]
  Relational Operator20/1 -> [VDHP_EAPS1NRMStable_flg]  "VDHP_EAPS1NRMStable_flg"
  VDHP_EPEDLIND_pct/1 -> [VDHP_EPEDLIND_pct]
  SR_Latch/1 -> AND/1
  NOT5/1 -> Timer1/2(reset)
  [VDHP_EAPS1NRMBase_pct] -> Add2/2
  [VDHP_EAPS2NRM_pct] -> Add3/1
  VDHP_EAPS2BAD_flg/1 -> [VDHP_EAPS2BAD_flg]
  VPMM_PowerSta_enum/1 -> [VPMM_PowerSta_enum]
  Timer1/1(time) -> Relational Operator20/1
  VDHP_EAPS2NRM_pct/1 -> [VDHP_EAPS2NRM_pct]
  Constant33/1 -> Relational Operator20/2
  [VDHP_EAPS1MINInit_pct] -> Switch20/3
  [VDHP_EAPS1MINMemValid_flg] -> Switch22/2
  Constant43/1 -> Switch22/3
  [VDHP_EAPS1MINMem_pct] -> Switch22/1
  Switch22/1 -> [VDHP_EAPS1MINInit_pct]  "VDHP_EAPS1MINInit_pct"
  [VDHP_EAPS2MINInit_pct] -> Switch5/3
  [VDHP_EAPS2MINMemValid_flg] -> Switch7/2
  Constant17/1 -> Switch7/3
  [VDHP_EAPS2MINMem_pct] -> Switch7/1
  Switch7/1 -> [VDHP_EAPS2MINInit_pct]  "VDHP_EAPS2MINInit_pct"
  VINP_EAPS2MINMem_pct/1 -> [VINP_EAPS2MINMem_pct]
  VINP_EAPS1MINMem_pct/1 -> [VINP_EAPS1MINMem_pct]
  [VINP_EAPS2MINMem_pct] -> [VDHP_EAPS2MINMem_pct]
  [VINP_EAPS1MINMem_pct] -> [VDHP_EAPS1MINMem_pct]
  Constant21/1 -> Add7/2
  [VDHP_EAPS1MINInit_pct] -> Add7/1
  Switch18/1 -> Max/1
  Max/1 -> Switch20/1
  [VDHP_EAPS1MIN_pct] -> Unit Delay2/1
  [VDHP_EAPS2MIN_pct] -> Unit Delay9/1
  Switch3/1 -> Max1/1
  Max1/1 -> Switch5/1
  Constant22/1 -> Add8/2
  [VDHP_EAPS2MINInit_pct] -> Add8/1
  Add8/1 -> Max1/2
  Add7/1 -> Max/2
  VINP_LVBattDet12V_V/1 -> [VINP_LVBattDet12V_V]
  VINP_CANMsgValidBMS5_flg/1 -> [VINP_CANMsgValidBMS5_flg]
  [VDHP_EAPS1LearnInRange_flg] -> AND2/1
  [VINP_LVBattDet12V_V] -> Relational Operator10/1, Relay/1
  Constant23/1 -> Relational Operator10/2
  Relay/1 -> AND5/1
  Relational Operator10/1 -> AND5/2
  [VINP_CANMsgValidBMS5_flg] -> AND5/3
  Constant24/1 -> Relational Operator11/2
  [VPMM_PowerSta_enum] -> Relational Operator11/1
  Constant26/1 -> Relational Operator14/2
  [VPMM_PowerSta_enum] -> Relational Operator14/1
  Relational Operator11/1 -> AND6/1
  Relational Operator14/1 -> AND6/2
  NOT/1 -> AND7/1
  NOT2/1 -> AND7/2
  Relational Operator12/1 -> AND8/1
  Relational Operator13/1 -> AND8/2
  Relational Operator/1 -> AND8/3
  Relational Operator1/1 -> AND8/4
  AND8/1 -> OR4/1
  AND5/1 -> OR4/3
  AND7/1 -> OR4/2
  AND6/1 -> OR4/4
  Relational Operator17/1 -> AND10/1
  Relational Operator18/1 -> AND10/2
  Constant29/1 -> Relational Operator18/2
  [VPMM_PowerSta_enum] -> Relational Operator18/1
  Constant27/1 -> Relational Operator16/2
  Constant28/1 -> Relational Operator17/2
  Relational Operator16/1 -> AND9/2
  [VINP_CANMsgValidBMS5_flg] -> AND9/3
  [VPMM_PowerSta_enum] -> Relational Operator17/1
  Relay1/1 -> AND9/1
  [VINP_LVBattDet12V_V] -> Relational Operator16/1, Relay1/1
  AND9/1 -> AND11/2
  AND10/1 -> AND11/3
  AND11/1 -> [VDHP_EAPSLearnUpEnable_flg]  "VDHP_EAPSLearnUpEnable_flg"
  [VDHP_EAPS2LearnInRange_flg] -> AND4/1
  Relational Operator27/1 -> AND13/1
  Relational Operator28/1 -> AND13/2
  Constant32/1 -> Relational Operator28/2
  [VPMM_PowerSta_enum] -> Relational Operator28/1
  Constant30/1 -> Relational Operator19/2
  Constant31/1 -> Relational Operator27/2
  Relational Operator19/1 -> AND12/2
  [VINP_CANMsgValidBMS5_flg] -> AND12/3
  [VPMM_PowerSta_enum] -> Relational Operator27/1
  Relay2/1 -> AND12/1
  [VINP_LVBattDet12V_V] -> Relational Operator19/1, Relay2/1
  NOT6/1 -> AND14/1
  NOT7/1 -> AND14/2
  Relational Operator7/1 -> AND15/1
  Relational Operator8/1 -> AND15/2
  Relational Operator6/1 -> AND15/4
  Relational Operator5/1 -> AND15/3
  AND14/1 -> OR1/2
  AND15/1 -> OR1/1
  AND12/1 -> OR1/3
  AND13/1 -> OR1/4
  VINP_ResetPedalZeroPosReq_enum/1 -> [VINP_ResetPedalZeroPosReq_enum]
  Constant34/1 -> Relational Operator29/2
  [VINP_ResetPedalZeroPosReq_enum] -> Relational Operator29/1
  Switch/1 -> [VDHP_EAPS1MIN_pct], VDHP_EAPS1MIN_pct/1  "VDHP_EAPS1MIN_pct"
  [VDHP_ResetPedalZeroPosStart_flg] -> Switch17/2
  Constant40/1 -> Switch/1
  Constant39/1 -> Switch/2
  Constant42/1 -> Switch17/1
  Switch17/1 -> Switch/3
  Constant44/1 -> Switch8/1
  [VDHP_ResetPedalZeroPosStart_flg] -> Switch8/2
  Switch5/1 -> Switch8/3
  Switch8/1 -> Switch2/3
  Relational Operator29/1 -> Latch/1
  Latch/1 -> VDHP_ResetPedalZeroPosStart_flg/1, [VDHP_ResetPedalZeroPosStart_flg]  "VDHP_ResetPedalZeroPosStart_flg"
  Latch2/1 -> Switch20/2  "VDHP_EAPS1Learned_flg"
  AND16/1 -> Latch2/1
  [VDHP_EAPS1LearnDwEnable_flg] -> AND16/1
  [VDHP_EAPSLearnUpEnable_flg] -> AND16/2
  [VDHP_EAPSLearnUpEnable_flg] -> AND17/2
  AND17/1 -> Latch1/1
  [VDHP_EAPS2LearnDwEnable_flg] -> AND17/1
  Max2/1 -> Switch18/1
  [VDHP_EAPS1NRM_pct] -> Max2/1
  Constant45/1 -> Max2/2
  Constant46/1 -> Max3/2
  Max3/1 -> Switch3/1
  [VDHP_EAPS2NRM_pct] -> Max3/1

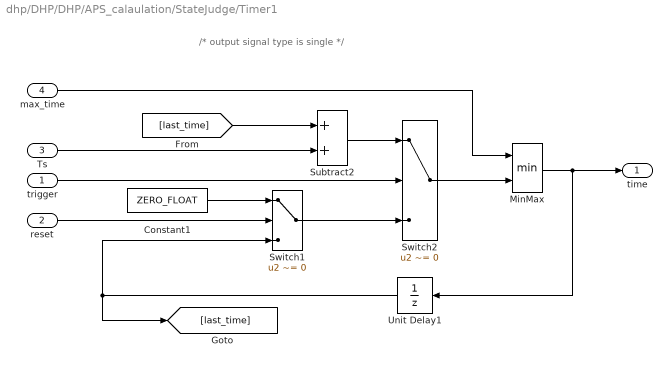
== system dhp/DHP/DHP/APS_calaulation/StateJudge/Timer1 ==
  note: /* output signal type is single */
  trigger : Inport
  reset : Inport  Port=2
  Ts : Inport  Port=3
  max_time : Inport  Port=4
  Constant1 : Constant  Value=ZERO_FLOAT  OutDataTypeStr=single
  MinMax : MinMax  Inputs=2
  Subtract2 : Sum
  Switch1 : Switch  Criteria=u2 ~= 0
      settings: AttributesFormatString=<%<Criteria>>
  Switch2 : Switch  Criteria=u2 ~= 0
      settings: AttributesFormatString=<%<Criteria>>
  Unit Delay1 : UnitDelay  SampleTime=-1  HasFrameUpgradeWarning=on
      settings: AttributesFormatString=<initial = %<X0>>
  time : Outport
  wires:
  [last_time] -> Subtract2/1
  max_time/1 -> MinMax/1
  Unit Delay1/1 -> [last_time], Switch1/3
  MinMax/1 -> Unit Delay1/1, time/1
  Switch2/1 -> MinMax/2
  Ts/1 -> Subtract2/2
  Switch1/1 -> Switch2/3
  Constant1/1 -> Switch1/1
  reset/1 -> Switch1/2
  trigger/1 -> Switch2/2
  Subtract2/1 -> Switch2/1

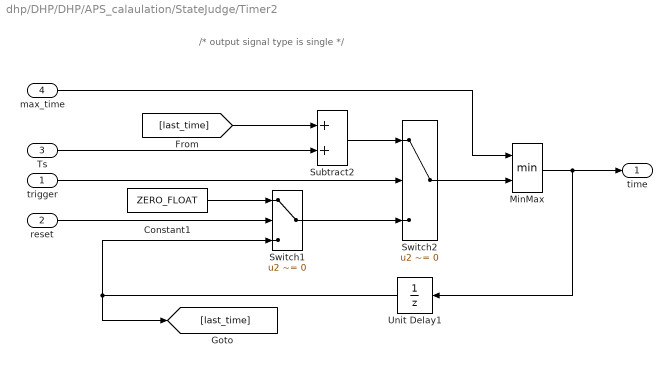
== system dhp/DHP/DHP/APS_calaulation/StateJudge/Timer2 ==
  note: /* output signal type is single */
  trigger : Inport
  reset : Inport  Port=2
  Ts : Inport  Port=3
  max_time : Inport  Port=4
  Constant1 : Constant  Value=ZERO_FLOAT  OutDataTypeStr=single
  MinMax : MinMax  Inputs=2
  Subtract2 : Sum
  Switch1 : Switch  Criteria=u2 ~= 0
      settings: AttributesFormatString=<%<Criteria>>
  Switch2 : Switch  Criteria=u2 ~= 0
      settings: AttributesFormatString=<%<Criteria>>
  Unit Delay1 : UnitDelay  SampleTime=-1  HasFrameUpgradeWarning=on
      settings: AttributesFormatString=<initial = %<X0>>
  time : Outport
  wires:
  Subtract2/1 -> Switch2/1
  trigger/1 -> Switch2/2
  reset/1 -> Switch1/2
  Constant1/1 -> Switch1/1
  Switch1/1 -> Switch2/3
  Ts/1 -> Subtract2/2
  Switch2/1 -> MinMax/2
  MinMax/1 -> time/1, Unit Delay1/1
  Unit Delay1/1 -> Switch1/3, [last_time]
  max_time/1 -> MinMax/1
  [last_time] -> Subtract2/1

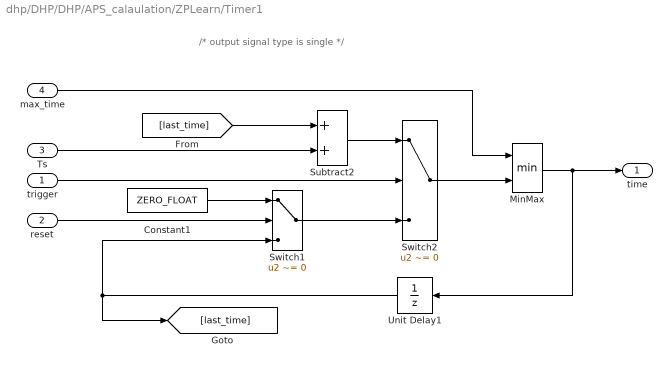
== system dhp/DHP/DHP/APS_calaulation/ZPLearn/Timer1 ==
  note: /* output signal type is single */
  trigger : Inport
  reset : Inport  Port=2
  Ts : Inport  Port=3
  max_time : Inport  Port=4
  Constant1 : Constant  Value=ZERO_FLOAT  OutDataTypeStr=single
  MinMax : MinMax  Inputs=2
  Subtract2 : Sum
  Switch1 : Switch  Criteria=u2 ~= 0
      settings: AttributesFormatString=<%<Criteria>>
  Switch2 : Switch  Criteria=u2 ~= 0
      settings: AttributesFormatString=<%<Criteria>>
  Unit Delay1 : UnitDelay  SampleTime=-1  HasFrameUpgradeWarning=on
      settings: AttributesFormatString=<initial = %<X0>>
  time : Outport
  wires:
  [last_time] -> Subtract2/1
  max_time/1 -> MinMax/1
  Unit Delay1/1 -> [last_time], Switch1/3
  MinMax/1 -> Unit Delay1/1, time/1
  Switch2/1 -> MinMax/2
  Ts/1 -> Subtract2/2
  Switch1/1 -> Switch2/3
  Constant1/1 -> Switch1/1
  reset/1 -> Switch1/2
  trigger/1 -> Switch2/2
  Subtract2/1 -> Switch2/1

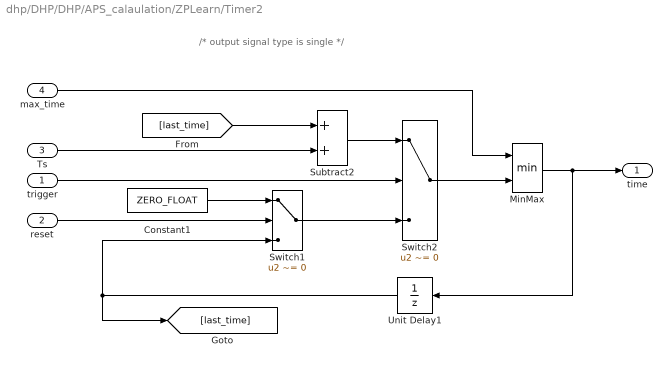
== system dhp/DHP/DHP/APS_calaulation/ZPLearn/Timer2 ==
  note: /* output signal type is single */
  trigger : Inport
  reset : Inport  Port=2
  Ts : Inport  Port=3
  max_time : Inport  Port=4
  Constant1 : Constant  Value=ZERO_FLOAT  OutDataTypeStr=single
  MinMax : MinMax  Inputs=2
  Subtract2 : Sum
  Switch1 : Switch  Criteria=u2 ~= 0
      settings: AttributesFormatString=<%<Criteria>>
  Switch2 : Switch  Criteria=u2 ~= 0
      settings: AttributesFormatString=<%<Criteria>>
  Unit Delay1 : UnitDelay  SampleTime=-1  HasFrameUpgradeWarning=on
      settings: AttributesFormatString=<initial = %<X0>>
  time : Outport
  wires:
  [last_time] -> Subtract2/1
  max_time/1 -> MinMax/1
  Unit Delay1/1 -> [last_time], Switch1/3
  MinMax/1 -> Unit Delay1/1, time/1
  Switch2/1 -> MinMax/2
  Ts/1 -> Subtract2/2
  Switch1/1 -> Switch2/3
  Constant1/1 -> Switch1/1
  reset/1 -> Switch1/2
  trigger/1 -> Switch2/2
  Subtract2/1 -> Switch2/1

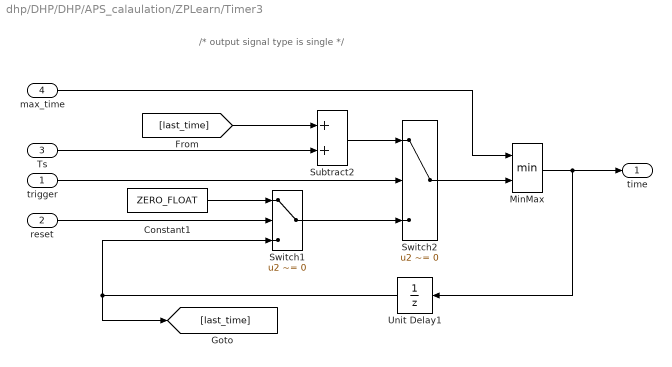
== system dhp/DHP/DHP/APS_calaulation/ZPLearn/Timer3 ==
  note: /* output signal type is single */
  trigger : Inport
  reset : Inport  Port=2
  Ts : Inport  Port=3
  max_time : Inport  Port=4
  Constant1 : Constant  Value=ZERO_FLOAT  OutDataTypeStr=single
  MinMax : MinMax  Inputs=2
  Subtract2 : Sum
  Switch1 : Switch  Criteria=u2 ~= 0
      settings: AttributesFormatString=<%<Criteria>>
  Switch2 : Switch  Criteria=u2 ~= 0
      settings: AttributesFormatString=<%<Criteria>>
  Unit Delay1 : UnitDelay  SampleTime=-1  HasFrameUpgradeWarning=on
      settings: AttributesFormatString=<initial = %<X0>>
  time : Outport
  wires:
  Subtract2/1 -> Switch2/1
  trigger/1 -> Switch2/2
  reset/1 -> Switch1/2
  Constant1/1 -> Switch1/1
  Switch1/1 -> Switch2/3
  Ts/1 -> Subtract2/2
  Switch2/1 -> MinMax/2
  MinMax/1 -> time/1, Unit Delay1/1
  Unit Delay1/1 -> Switch1/3, [last_time]
  max_time/1 -> MinMax/1
  [last_time] -> Subtract2/1

== system dhp/DHP/DHP/APS_calaulation/ZPLearn/Timer4 ==
  note: /* output signal type is single */
  trigger : Inport
  reset : Inport  Port=2
  Ts : Inport  Port=3
  max_time : Inport  Port=4
  Constant1 : Constant  Value=ZERO_FLOAT  OutDataTypeStr=single
  MinMax : MinMax  Inputs=2
  Subtract2 : Sum
  Switch1 : Switch  Criteria=u2 ~= 0
      settings: AttributesFormatString=<%<Criteria>>
  Switch2 : Switch  Criteria=u2 ~= 0
      settings: AttributesFormatString=<%<Criteria>>
  Unit Delay1 : UnitDelay  SampleTime=-1  HasFrameUpgradeWarning=on
      settings: AttributesFormatString=<initial = %<X0>>
  time : Outport
  wires:
  Subtract2/1 -> Switch2/1
  trigger/1 -> Switch2/2
  reset/1 -> Switch1/2
  Constant1/1 -> Switch1/1
  Switch1/1 -> Switch2/3
  Ts/1 -> Subtract2/2
  Switch2/1 -> MinMax/2
  MinMax/1 -> time/1, Unit Delay1/1
  Unit Delay1/1 -> Switch1/3, [last_time]
  max_time/1 -> MinMax/1
  [last_time] -> Subtract2/1
